simulink model "FM_V6_Zikun"  (R2022b)
settings: Solver=VariableStepAuto  StartTime=0.0  StopTime=1240
values from neighbouring files (symbols this model uses):
  A_fc = 550    [CNV.m]
  A_st = 1.1*A_fc*1E-4*n_cell*0.0012    (= 0.047553)    [CNV.m]
  A_T_rm = 0.005    [CNV.m]
  b11 = 0.005139    [CNV.m]
  b12 = 0.00326    [CNV.m]
  b2 = 350    [CNV.m]
  c1 = 10    [CNV.m]
  c3 = 2    [CNV.m]
  cc = 30    [CNV.m]
  Cd_rm = 0.0124    [CNV.m]
  Cp_air = 1005    [CNV.m]
  Cp_cl = 4180    [CNV.m]
  Cp_st = Cp_Al*1.5    (= 1350)    [CNV.m]
  F = 96485    [CNV.m]
  gamma = 1.4    [CNV.m]
  H_conv_st = 3    [CNV.m]
  i_max = 2.2    [CNV.m]
  k_ca_out = 0.2177*10^(-5)    (= 2.177e-06)    [CNV.m]
  K_sm_out = 0.3629*10^-5    (= 3.629e-06)    [CNV.m]
  kd_cp = 0.01    [CNV.m]
  kd_rm = 0    [CNV.m]
  ki_cp = 0.1    [CNV.m]
  ki_fan = -1E-5    (= -1e-05)    [CNV.m]
  ki_rm = -5E-8    (= -5e-08)    [CNV.m]
  kp_cp = 7.5    [CNV.m]
  kp_fan = -0.5    [CNV.m]
  kp_rm = -8E-7    (= -8e-07)    [CNV.m]
  M_a = 29*10^-3    (= 0.029)    [CNV.m]
  M_H2 = 2*10^-3    (= 0.002)    [CNV.m]
  m_H2_initial = P_atm*V_an/(R_H2*T_atm)    (= 0.00044494386048)    [CNV.m]
  m_H2O_initial = 0.005    [CNV.m]
  M_m_dry = 1.1    [CNV.m]
  M_N2 = 28*10^-3    (= 0.028)    [CNV.m]
  m_N2_initial = P_atm*(1-y_O2)*V_ca/(R_N2*T_atm)    (= 0.00586138039643)    [CNV.m]
  M_O2 = 32*10^-3    (= 0.032)    [CNV.m]
  m_O2_initial = P_atm*y_O2*V_ca/(R_O2*T_atm)    (= 0.00177998712422)    [CNV.m]
  m_st = n_cell*A_fc*t_m*rho_m_dry+(V_ca+V_an)*rho_Al*2.5    (= 87.4506875)    [CNV.m]
  M_v = 18*10^-3    (= 0.018)    [CNV.m]
  n_cell = 655    [CNV.m]
  P_a = P_atm*(1-L*h/T_atm)^(g*M_a/(R*L))    [CNV.m]
  P_atm = 101.25*10^3    (= 101250)    [CNV.m]
  P_ca_ref = 2.5*P_a    [CNV.m]
  phi_a = 0.1    [CNV.m]
  phi_des = 1    [CNV.m]
  R = 8.315    [CNV.m]
  R_a = 286.9    [CNV.m]
  R_H2 = 4124.3    [CNV.m]
  R_N2 = 296.8    [CNV.m]
  R_O2 = 259.8    [CNV.m]
  R_v = 461.5    [CNV.m]
  rho_a = P_a/(R_a*T_a)    [CNV.m]
  rho_H2 = 0.0899    [CNV.m]
  rho_m_dry = 0.002    [CNV.m]
  rho_N2 = 1.165    [CNV.m]
  T_a = T_atm-h*L    [CNV.m]
  T_atm = 298.15    [CNV.m]
  T_cl = 353.15    [CNV.m]
  t_m = 0.01    [CNV.m]
  T_rm = 303.15    [CNV.m]
  T_st_ref = 353.15    [CNV.m]
  V_an = n_cell*A_fc*10^(-4)*0.0005*0.3    (= 0.00540375)    [CNV.m]
  V_ca = n_cell*A_fc*10^(-4)*0.0006*0.3    (= 0.0064845)    [CNV.m]
  V_rm = 0.005    [CNV.m]
  V_sm = 0.02    [CNV.m]
  y_O2_ca_in = 0.21    [CNV.m]
libraries: fl_lib x64, nesl_utility x40, ee_lib x18, fl_ps_legacy_lib x6, SimscapeFluids_lib x5, slpidlib x4, simulink x3, batteryecm_lib x1, autolibshared x1
(part 4 of 6)

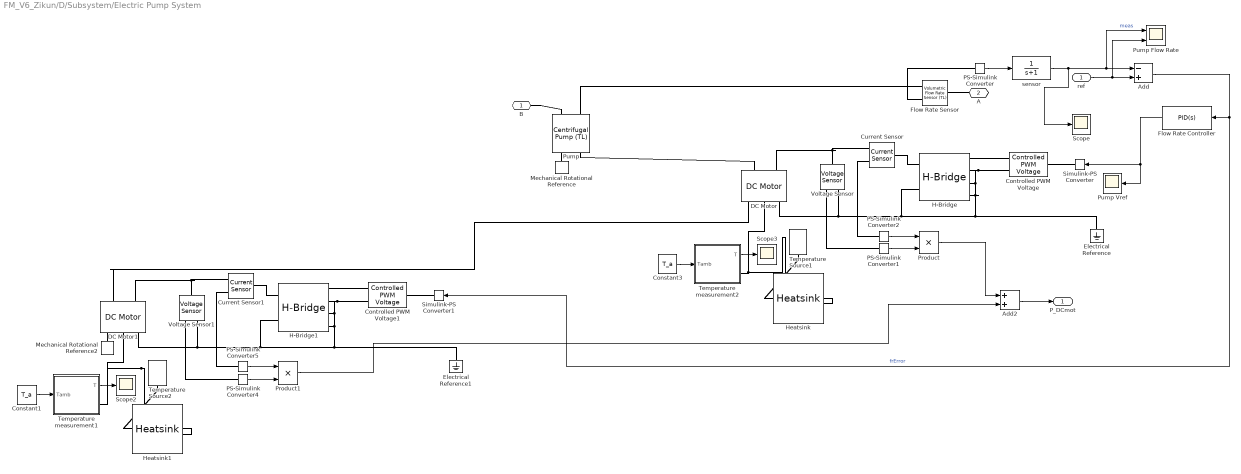
== system FM_V6_Zikun/D/Subsystem/Electric Pump System ==
  ref : Inport
  Add : Sum  Inputs=-+
  Add2 : Sum
  Constant1 : Constant  Value=T_a
  Constant3 : Constant  Value=T_a
  Controlled PWM Voltage : ee_lib/Integrated Circuits/Controlled PWM Voltage  F=4000 Hz  TD=0 s  pulse_width_offset=0 s  pulse_min=0 s  pwm_or_av=2  event_type=1  sample_time=5e-6 s  Vmin=0 V  Vmax=5 V  Vm=5 V  u_min=0  u_max=5
      settings: InternalSimscapePortConfiguration="{\"Bottom\":[],\"Left\":[{\"id\":\"u\",\"label\":\"u\",\"type\":\"input\"}],\"Right\":[{\"id\":\"p2\",\"label\":\"PWM\",\"type\":\"foundation.electrical.electrical\"},{\"id\":\"n2\",\"label\":\"REF\",\"type\":\"foundation.electrical.electrical\"}],\"Top\":[]}"
  Controlled PWM Voltage1 : ee_lib/Integrated Circuits/Controlled PWM Voltage  F=4000 Hz  TD=0 s  pulse_width_offset=0 s  pulse_min=0 s  pwm_or_av=2  event_type=1  sample_time=5e-6 s  Vmin=0 V  Vmax=5 V  Vm=5 V  u_min=0  u_max=5
      settings: InternalSimscapePortConfiguration="{\"Bottom\":[],\"Left\":[{\"id\":\"u\",\"label\":\"u\",\"type\":\"input\"}],\"Right\":[{\"id\":\"p2\",\"label\":\"PWM\",\"type\":\"foundation.electrical.electrical\"},{\"id\":\"n2\",\"label\":\"REF\",\"type\":\"foundation.electrical.electrical\"}],\"Top\":[]}"
  Current Sensor : fl_lib/Electrical/Electrical Sensors/Current Sensor
  Current Sensor1 : fl_lib/Electrical/Electrical Sensors/Current Sensor
  DC Motor : ee_lib/Electromechanical/Brushed Motors/DC Motor  Tag={'toolbox/physmod/elec/library/m/ee_lib_parts';'Electromechanical/Brushed_Motors/DC_Motor/Maxon/RE_65_388988_60.xml'}  field_option=ee.enum.field_option.pm  Rf=100 % Parameter not set Ohm  Lf=1 % Parameter not set H  Laf=0.15 % Parameter not set H  If0=0 % Parameter not set A  parameterization=ee.enum.dcparam_option.circuit_param  Ra=0.568 Ohm  La=0.251 mH  emf_or_torque=ee.enum.emf_or_torque.kv  Kv=16.05136 mV/rpm  Ki=153.27924 % Parameter estimated mN*m/A  T_stall=0.24e-3 % Parameter not set N*m  w_max=19100 % Parameter not set rpm  w_rated=15000 % Parameter not set rpm  P_rated=0.08 % Parameter not set W  V_rated=1.5 % Parameter not set V  lam_param=ee.enum.lam_param.current  i_noload=0.231 A  V_i_noload=60 V  J=1320 g*cm^2  lam=0 % % Parameter not set mN*m/(rad/s)  speed0=0 % Parameter not set rpm  enable_fault_armature=simscape.enum.onoff.off  rev_faulted=1 / 3 % Parameter not set  G_faulted_armature=1e-5 % Parameter not set S  fault_trigger_armature=ee.enum.faults.faultTrigger.temporal  t_fault_armature=1 % Parameter not set s  max_permissible_current_armature=inf % Parameter not set A  t_fail_on_current_armature=1 % Parameter not set s  enable_fault_field=simscape.enum.onoff.off  G_faulted_field=1e-5 % Parameter not set S  fault_trigger_field=ee.enum.faults.faultTrigger.temporal  t_fault_field=1 % Parameter not set s  max_permissible_current_field=inf % Parameter not set A  t_fail_on_current_field=1 % Parameter not set s  fault_action=simscape.enum.assert.action.none  alpha=3.93e-3 % Parameter not set 1/K  Tmeas=25 % Parameter not set degC  thermal_mass=667.588357588358 % Parameter estimated J/K  initial_temperature=25 % Parameter not set degC
      settings: AttributesFormatString=Maxon:RE_65_388988_60  InternalSimscapePortConfiguration="{\"Bottom\":[],\"Left\":[{\"id\":\"p\",\"label\":\"+\",\"type\":\"foundation.electrical.electrical\"},{\"id\":\"R\",\"label\":\"R\",\"type\":\"foundation.mechanical.rotational.rotational\"}],\"Right\":[{\"id\":\"n\",\"label\":\"-\",\"type\":\"foundation.electrical.electrical\"},{\"id\":\"H\",\"label\":\"H\",\"type\":\"foundation.thermal.thermal\"},{\"id\":\"C\",\"label\":\"C\",\"type\":\"foundation.mechanical.rotational.rotational\"}],\"Top\":[]}"
  DC Motor1 : ee_lib/Electromechanical/Brushed Motors/DC Motor  Tag={'toolbox/physmod/elec/library/m/ee_lib_parts';'Electromechanical/Brushed_Motors/DC_Motor/Maxon/RE_65_388988_60.xml'}  field_option=ee.enum.field_option.pm  Rf=100 % Parameter not set Ohm  Lf=1 % Parameter not set H  Laf=0.15 % Parameter not set H  If0=0 % Parameter not set A  parameterization=ee.enum.dcparam_option.circuit_param  Ra=0.568 Ohm  La=0.251 mH  emf_or_torque=ee.enum.emf_or_torque.kv  Kv=16.05136 mV/rpm  Ki=153.27924 % Parameter estimated mN*m/A  T_stall=0.24e-3 % Parameter not set N*m  w_max=19100 % Parameter not set rpm  w_rated=15000 % Parameter not set rpm  P_rated=0.08 % Parameter not set W  V_rated=1.5 % Parameter not set V  lam_param=ee.enum.lam_param.current  i_noload=0.231 A  V_i_noload=60 V  J=1320 g*cm^2  lam=0 % % Parameter not set mN*m/(rad/s)  speed0=0 % Parameter not set rpm  enable_fault_armature=simscape.enum.onoff.off  rev_faulted=1 / 3 % Parameter not set  G_faulted_armature=1e-5 % Parameter not set S  fault_trigger_armature=ee.enum.faults.faultTrigger.temporal  t_fault_armature=1 % Parameter not set s  max_permissible_current_armature=inf % Parameter not set A  t_fail_on_current_armature=1 % Parameter not set s  enable_fault_field=simscape.enum.onoff.off  G_faulted_field=1e-5 % Parameter not set S  fault_trigger_field=ee.enum.faults.faultTrigger.temporal  t_fault_field=1 % Parameter not set s  max_permissible_current_field=inf % Parameter not set A  t_fail_on_current_field=1 % Parameter not set s  fault_action=simscape.enum.assert.action.none  alpha=3.93e-3 % Parameter not set 1/K  Tmeas=25 % Parameter not set degC  thermal_mass=667.588357588358 % Parameter estimated J/K  initial_temperature=25 % Parameter not set degC
      settings: AttributesFormatString=Maxon:RE_65_388988_60  InternalSimscapePortConfiguration="{\"Bottom\":[],\"Left\":[{\"id\":\"p\",\"label\":\"+\",\"type\":\"foundation.electrical.electrical\"},{\"id\":\"R\",\"label\":\"R\",\"type\":\"foundation.mechanical.rotational.rotational\"}],\"Right\":[{\"id\":\"n\",\"label\":\"-\",\"type\":\"foundation.electrical.electrical\"},{\"id\":\"H\",\"label\":\"H\",\"type\":\"foundation.thermal.thermal\"},{\"id\":\"C\",\"label\":\"C\",\"type\":\"foundation.mechanical.rotational.rotational\"}],\"Top\":[]}"
  Electrical Reference : fl_lib/Electrical/Electrical Elements/Electrical Reference
  Electrical Reference1 : fl_lib/Electrical/Electrical Elements/Electrical Reference
  Flow Rate Sensor : fl_lib/Thermal Liquid/Sensors/Volumetric Flow Rate Sensor (TL)
      settings: InternalSimscapePortConfiguration="{\"Bottom\":[],\"Left\":[{\"id\":\"A\",\"label\":\"A\",\"type\":\"foundation.thermal_liquid.thermal_liquid\"}],\"Right\":[{\"id\":\"B\",\"label\":\"B\",\"type\":\"foundation.thermal_liquid.thermal_liquid\"},{\"id\":\"V\",\"label\":\"V\",\"type\":\"output\"}],\"Top\":[]}"
  Flow Rate Controller : slpidlib/PID Controller  Controller=PID  Form=Parallel  TimeDomain=Continuous-time  UseExternalTs=off  SampleTime=-1  IntegratorMethod=Forward Euler  FilterMethod=Forward Euler  ControllerParametersSource=internal  P=1  I=5e-1  UseKiTs=off  D=0  N=10  UseFilter=on  TunerSelectOption=Transfer Function Based (PID Tuner App)  ZeroCross=off  InitialConditionSource=internal  InitialConditionForIntegrator=0  InitialConditionForFilter=0  DifferentiatorICPrevScaledInput=0  ExternalReset=none  TrackingMode=off  Kt=1  LimitOutput=on  SatLimitsSource=internal  UpperSaturationLimit=5  LowerSaturationLimit=0  LinearizeAsGain=on  AntiWindupMode=none  Kb=1  LimitIntegrator=off  UpperIntegratorSaturationLimit=inf  LowerIntegratorSaturationLimit=-inf  POutMin=[]  POutMax=[]  IOutMin=[]  IOutMax=[]  DOutMin=[]  DOutMax=[]  NOutMin=[]  NOutMax=[]  SumOutMin=[]  SumOutMax=[]  SaturationOutMin=[]  SaturationOutMax=[]  PParamMin=[]  PParamMax=[]  IParamMin=[]  IParamMax=[]  DParamMin=[]  DParamMax=[]  NParamMin=[]  NParamMax=[]  KbParamMin=[]  KbParamMax=[]  KtParamMin=[]  KtParamMax=[]  KbOutMin=[]  KbOutMax=[]  KtOutMin=[]  KtOutMax=[]  IntegratorOutMin=[]  IntegratorOutMax=[]  FilterOutMin=[]  FilterOutMax=[]  SumI1OutMin=[]  SumI1OutMax=[]  SumI2OutMin=[]  SumI2OutMax=[]  SumI3OutMin=[]  SumI3OutMax=[]  SumI4OutMin=[]  SumI4OutMax=[]  SumDOutMin=[]  SumDOutMax=[]  DifferentiatorOutMin=[]  DifferentiatorOutMax=[]  FilterDiffOutCoefMin=[]  FilterDiffOutCoefMax=[]  ReciprocalOutMin=[]  ReciprocalOutMax=[]  SumDenOutMin=[]  SumDenOutMax=[]  SumNumOutMin=[]  SumNumOutMax=[]  DivideOutMin=[]  DivideOutMax=[]  UdiffTsProdOutMin=[]  UdiffTsProdOutMax=[]  NTsProdOutMin=[]  NTsProdOutMax=[]  UintegralTsProdOutMin=[]  UintegralTsProdOutMax=[]  UngainTsProdOutMin=[]  UngainTsProdOutMax=[]  ClampingZeroOutDataTypeStr=Inherit: Inherit via back propagation  ClampingZeroOutMin=[]  ClampingZeroOutMax=[]  FilterDenConstantOutDataTypeStr=Inherit: Inherit via back propagation  FilterDenConstantOutMin=[]  FilterDenConstantOutMax=[]  PCopyOutDataTypeStr=Inherit: Inherit via back propagation  PCopyOutMin=[]  PCopyOutMax=[]  NCopyOutDataTypeStr=Inherit: Inherit via back propagation  NCopyOutMin=[]  NCopyOutMax=[]  IntegratorContinuousStateAttributes=''  IntegratorStateMustResolveToSignalObject=off  IntegratorRTWStateStorageClass=Auto  FilterContinuousStateAttributes=''  FilterStateMustResolveToSignalObject=off  FilterRTWStateStorageClass=Auto  ParallelPVariant=InternalParameters  IdealPVariant=Disabled  IVariant=InternalParameters  DVariant=InternalParameters  IntegratorVariant=Continuous  SatVariant=Enabled  AWVariant=Passthrough  PCopyVariant=Disabled  TRVariant=Disabled  FdbkBlocksVariant=Forward  IdealPFdbkVariant=Disabled  SatFdbkVariant=Disabled  DerivativeFilterVariant=ContFilter  NVariant=InternalParameters  NCopyVariant=Disabled  FilterICVariant=InternalICsFilter  IntegratorICVariant=InternalICs  ExternalResetVariant=Disabled  TRSumVariant=Passthrough  SumFdbkVariant=Disabled  SumVariant=Sum_PID  TsampFilterVariant=InternalTs  TsampNgainVariant=Passthrough  TsampIntegralVariant=Passthrough  ExternalSaturationOutDataTypeStr=Inherit: Same as second input
  H-Bridge : ee_lib/Semiconductors & Converters/Converters/H-Bridge  supply_ports=ee.enum.supply_ports.hidesupply  pwm_or_av=2  regenerative_braking_mode=2  discontinuous=0  freewheeling_mode=1  Rload=3.38+0.1 Ohm  Lload=1e-5 H  F=4 kHz  Venable=2.5 V  Vmax=5 V  Vreverse=2.5 V  Vbrake=2.5 V  Vm=12 V  Ron=0.1 Ohm  Don=0.1 Ohm  Goff=1e-6 S  Tmeas=298.15 K  Ron2=0.1 Ohm  Don2=0.05 Ohm  Tmeas2=398.15 K  thermal_mass=100 J/K  initial_temperature=298.15 K
  H-Bridge1 : ee_lib/Semiconductors & Converters/Converters/H-Bridge  supply_ports=ee.enum.supply_ports.hidesupply  pwm_or_av=2  regenerative_braking_mode=2  discontinuous=0  freewheeling_mode=1  Rload=3.38+0.1 Ohm  Lload=1e-5 H  F=4 kHz  Venable=2.5 V  Vmax=5 V  Vreverse=2.5 V  Vbrake=2.5 V  Vm=12 V  Ron=0.1 Ohm  Don=0.1 Ohm  Goff=1e-6 S  Tmeas=298.15 K  Ron2=0.1 Ohm  Don2=0.05 Ohm  Tmeas2=398.15 K  thermal_mass=100 J/K  initial_temperature=298.15 K
  Heatsink : ee_lib/Passive/Thermal/Heatsink  parameterization=ee.enum.passive.thermal.heatsinkParam.rectangularFin  convection=ee.enum.passive.thermal.heatsinkConvection.natural  T_vec_Q=[10, 30, 50, 70, 90] K  v_vec_Q=[0, 1, 2, 3] m/s  Q_TLU1=[6.1, 23.6, 44.5, 67.5, 92.3] W  Q_TLU2=[6.1, 18.8, 22.8, 25.7; 23.6, 61.1, 73, 81.5; 44.5, 106.4, 125.9, 140.1; 67.5, 153.5, 180.7, 200.3; 92.3, 202.1, 236.9, 262] W  T_vec_h=[10, 30, 50, 70, 90] K  v_vec_h=[0, 1, 2, 3] m/s  h_TLU1=[5.4, 7.02, 7.98, 8.68, 9.26] W/(K*m^2)  h_TLU2=[5.4, 17.86, 22.17, 25.41; 7.02, 19.49, 23.8, 27.03; 7.97, 20.44, 24.75, 27.99; 8.68, 21.15, 25.46, 28.69; 9.26, 21.73, 26.04, 29.27] W/(K*m^2)  h_vec=[5, 10, 15, 20, 25, 30] W/(K*m^2)  eff_TLU=[96.97, 94.16, 91.53, 89.08, 86.78, 84.62]  height=0.1 m  thick=6.5e-4 m  depth=0.4 m  gap=9.4e-3 m  num_fins=100  k_fin=500 W/(K*m)  A_total=0.1171 m^2  nu=1.51e-5 m^2/s  alpha=2.07e-5 m^2/s  k_fluid=25e-3 W/(K*m)  beta=3.3e-3 1/K  mass=13 kg  sp_heat=550 J/(K*kg)  T_hs_specify=off  T_hs_priority=High  T_hs=300 K  T_hs_nominal_specify=off  T_hs_nominal_unit=K  T_hs_nominal_value=1  Q_A_specify=off  Q_A_priority=None  Q_A=0 W  Q_A_nominal_specify=off  Q_A_nominal_unit=W  Q_A_nominal_value=1  Q_C_specify=off  Q_C_priority=None  Q_C=0 W  Q_C_nominal_specify=off  Q_C_nominal_unit=W  Q_C_nominal_value=1
      settings: InternalSimscapePortConfiguration="{\"Bottom\":[{\"id\":\"C\",\"label\":\"C\",\"type\":\"foundation.thermal.thermal\"}],\"Left\":[],\"Right\":[],\"Top\":[{\"id\":\"A\",\"label\":\"A\",\"type\":\"foundation.thermal.thermal\"}]}"
  Heatsink1 : ee_lib/Passive/Thermal/Heatsink  parameterization=ee.enum.passive.thermal.heatsinkParam.rectangularFin  convection=ee.enum.passive.thermal.heatsinkConvection.natural  T_vec_Q=[10, 30, 50, 70, 90] K  v_vec_Q=[0, 1, 2, 3] m/s  Q_TLU1=[6.1, 23.6, 44.5, 67.5, 92.3] W  Q_TLU2=[6.1, 18.8, 22.8, 25.7; 23.6, 61.1, 73, 81.5; 44.5, 106.4, 125.9, 140.1; 67.5, 153.5, 180.7, 200.3; 92.3, 202.1, 236.9, 262] W  T_vec_h=[10, 30, 50, 70, 90] K  v_vec_h=[0, 1, 2, 3] m/s  h_TLU1=[5.4, 7.02, 7.98, 8.68, 9.26] W/(K*m^2)  h_TLU2=[5.4, 17.86, 22.17, 25.41; 7.02, 19.49, 23.8, 27.03; 7.97, 20.44, 24.75, 27.99; 8.68, 21.15, 25.46, 28.69; 9.26, 21.73, 26.04, 29.27] W/(K*m^2)  h_vec=[5, 10, 15, 20, 25, 30] W/(K*m^2)  eff_TLU=[96.97, 94.16, 91.53, 89.08, 86.78, 84.62]  height=0.1 m  thick=6.5e-4 m  depth=0.4 m  gap=9.4e-3 m  num_fins=100  k_fin=500 W/(K*m)  A_total=0.1171 m^2  nu=1.51e-5 m^2/s  alpha=2.07e-5 m^2/s  k_fluid=25e-3 W/(K*m)  beta=3.3e-3 1/K  mass=13 kg  sp_heat=550 J/(K*kg)  T_hs_specify=off  T_hs_priority=High  T_hs=300 K  T_hs_nominal_specify=off  T_hs_nominal_unit=K  T_hs_nominal_value=1  Q_A_specify=off  Q_A_priority=None  Q_A=0 W  Q_A_nominal_specify=off  Q_A_nominal_unit=W  Q_A_nominal_value=1  Q_C_specify=off  Q_C_priority=None  Q_C=0 W  Q_C_nominal_specify=off  Q_C_nominal_unit=W  Q_C_nominal_value=1
      settings: InternalSimscapePortConfiguration="{\"Bottom\":[{\"id\":\"C\",\"label\":\"C\",\"type\":\"foundation.thermal.thermal\"}],\"Left\":[],\"Right\":[],\"Top\":[{\"id\":\"A\",\"label\":\"A\",\"type\":\"foundation.thermal.thermal\"}]}"
  Mechanical Rotational Reference : fl_lib/Mechanical/Rotational Elements/Mechanical Rotational Reference
  Mechanical Rotational Reference2 : fl_lib/Mechanical/Rotational Elements/Mechanical Rotational Reference
  PS-Simulink Converter : nesl_utility/PS-Simulink Converter  PhysicalDomain=network_engine_domain  SubClassName=ps_output  LeftPortType=input  RightPortType=output  PseudoPeriodic=off  Frequencies=[]  VectorFormat=inherit  Unit=lpm  AffineConversion=off
  PS-Simulink Converter{1..2,4..5} (4 alike) : nesl_utility/PS-Simulink Converter  PhysicalDomain=network_engine_domain  SubClassName=ps_output  LeftPortType=input  RightPortType=output  PseudoPeriodic=off  Frequencies=[]  VectorFormat=inherit  Unit=inherit  AffineConversion=off
  Product : Product
  Product1 : Product
  Pump : SimscapeFluids_lib/Thermal Liquid/Pumps & Motors/Centrifugal Pump (TL)  pump_parameterization=fluids.thermal_liquid.pumps_motors.enum.CentrifugalPumpParameterization.Table1D  capacity_ref_nominal=7 lpm  head_ref_nominal=3 m  power_ref_nominal=5 W  head_ref_max=4 m  capacity_ref_max=12 lpm  omega_ref_analytic=4000 rpm  flow_rate_1D_TLU=[16.67, 30, 40, 53.33, 66.67, 83.33] lpm  head_1D_TLU=[50, 47.5, 45, 40, 35, 25] m  power_1D_TLU=[.6, .75, .85, .93, .98, .99] kW  omega_ref_1D=3500 rpm  rho_ref_1D=998.21 kg/m^3  flow_rate_2D_TLU=[16.67, 23.33, 30, 40, 53.33, 60] lpm  omega_2D_TLU=[2450, 2800, 3150, 3500] rpm  head_2D_TLU=[25, 32.7, 42.5, 50; 24, 31.7, 41, 49; 22.7, 30.5, 39, 47.5; 20, 28, 36, 45; 15.7, 24, 32, 40; 12.5, 21, 29.5, 37.5] m  power_2D_TLU=[.28, .38, .5, .6; .31, .41, .55, .68; .33, .44, .6, .75; .36, .48, .65, .83; .38, .53, .72, .93; .39, .55, .75, .97] kW  rho_ref_2D=998.21 kg/m^3  diameter_ratio=1  mech_orientation=fluids.thermal_liquid.pumps_motors.enum.CentrifugalPumpMechOrientation.Positive  area=0.03^2*pi/4 m^2
      settings: InternalSimscapePortConfiguration="{\"Bottom\":[],\"Left\":[{\"id\":\"A\",\"label\":\"A\",\"type\":\"foundation.thermal_liquid.thermal_liquid\"},{\"id\":\"B\",\"label\":\"B\",\"type\":\"foundation.thermal_liquid.thermal_liquid\"}],\"Right\":[{\"id\":\"R\",\"label\":\"R\",\"type\":\"foundation.mechanical.rotational.rotational\"},{\"id\":\"C\",\"label\":\"C\",\"type\":\"foundation.mechanical.rotational.rotational\"}],\"Top\":[]}"
  Pump Flow Rate : Scope  NumInputPorts=2
  Pump Vref : Scope
  Scope : Scope
  Scope2 : Scope
  Scope3 : Scope
  Simulink-PS Converter : nesl_utility/Simulink-PS Converter  PhysicalDomain=network_engine_domain  SubClassName=ps_input  LeftPortType=input  RightPortType=output  PseudoPeriodic=off  Frequencies=[]  NoiseDistribution=none  NoiseParameters=[]  Unit=1  AffineConversion=off  FilteringAndDerivatives=provide  SimscapeFilterOrder=1  InputFilterTimeConstant=0.001  UdotUserProvided=0
  Simulink-PS Converter1 : nesl_utility/Simulink-PS Converter  PhysicalDomain=network_engine_domain  SubClassName=ps_input  LeftPortType=input  RightPortType=output  PseudoPeriodic=off  Frequencies=[]  NoiseDistribution=none  NoiseParameters=[]  Unit=1  AffineConversion=off  FilteringAndDerivatives=provide  SimscapeFilterOrder=1  InputFilterTimeConstant=0.001  UdotUserProvided=0
  Temperature measurement1 : Subsystem
  Temperature measurement2 : Subsystem
  Temperature Source1 : fl_lib/Thermal/Thermal Sources/Temperature Source  temperature=T_a K
  Temperature Source2 : fl_lib/Thermal/Thermal Sources/Temperature Source  temperature=T_a K
  Voltage Sensor : fl_lib/Electrical/Electrical Sensors/Voltage Sensor
  Voltage Sensor1 : fl_lib/Electrical/Electrical Sensors/Voltage Sensor
  sensor : TransferFcn  Denominator=[1, 1]
  B : PMIOPort  Side=Left
  A : PMIOPort  Port=2  Side=Left
  P_DCmot : Outport
  wires:
  Flow Rate Controller/1 -> Pump Vref/1, Simulink-PS Converter/1
  Add/1 -> Simulink-PS Converter1/1, Flow Rate Controller/1  "frError"
  PS-Simulink Converter/1 -> sensor/1
  sensor/1 -> Scope/1, Pump Flow Rate/1, Add/1  "meas"
  PS-Simulink Converter2/1 -> Product/1
  PS-Simulink Converter1/1 -> Product/2
  Product/1 -> Add2/1
  Temperature measurement2/1(T) -> Scope3/1
  Constant3/1 -> Temperature measurement2/1(Tamb)
  Product1/1 -> Add2/2
  PS-Simulink Converter4/1 -> Product1/2
  Temperature measurement1/1(T) -> Scope2/1
  ref/1 -> Pump Flow Rate/2, Add/2
  PS-Simulink Converter5/1 -> Product1/1
  Constant1/1 -> Temperature measurement1/1(Tamb)
  Add2/1 -> P_DCmot/1
  connections:
  Mechanical Rotational Reference/LConn1 -- Pump/RConn2
  DC Motor/LConn2 -- Pump/RConn1
  B/RConn1 -- Pump/LConn2
  H-Bridge/LConn4 -- Controlled PWM Voltage/RConn2 -- H-Bridge/LConn2 -- H-Bridge/LConn3 -- DC Motor/RConn1 -- Voltage Sensor/RConn2 -- H-Bridge/RConn2 -- Electrical Reference/LConn1
  H-Bridge/LConn1 -- Controlled PWM Voltage/RConn1
  Voltage Sensor/LConn1 -- DC Motor/LConn1 -- Current Sensor/RConn2
  Flow Rate Sensor/LConn1 -- A/RConn1
  Flow Rate Sensor/RConn1 -- Pump/LConn1
  Flow Rate Sensor/RConn2 -- PS-Simulink Converter/LConn1
  Simulink-PS Converter/RConn1 -- Controlled PWM Voltage/LConn1
  PS-Simulink Converter1/LConn1 -- Voltage Sensor/RConn1
  PS-Simulink Converter2/LConn1 -- Current Sensor/RConn1
  Current Sensor/LConn1 -- H-Bridge/RConn1
  DC Motor/RConn3 -- DC Motor1/LConn2
  Temperature measurement2/RConn1 -- DC Motor/RConn2 -- Heatsink/RConn1
  Heatsink/LConn1 -- Temperature Source1/LConn1
  Current Sensor1/RConn2 -- Voltage Sensor1/LConn1 -- DC Motor1/LConn1
  Heatsink1/RConn1 -- Temperature measurement1/RConn1 -- DC Motor1/RConn2
  H-Bridge1/LConn2 -- H-Bridge1/LConn4 -- DC Motor1/RConn1 -- Voltage Sensor1/RConn2 -- H-Bridge1/RConn2 -- Electrical Reference1/LConn1 -- H-Bridge1/LConn3 -- Controlled PWM Voltage1/RConn2
  Heatsink1/LConn1 -- Temperature Source2/LConn1
  Simulink-PS Converter1/RConn1 -- Controlled PWM Voltage1/LConn1
  PS-Simulink Converter4/LConn1 -- Voltage Sensor1/RConn1
  Current Sensor1/LConn1 -- H-Bridge1/RConn1
  PS-Simulink Converter5/LConn1 -- Current Sensor1/RConn1
  H-Bridge1/LConn1 -- Controlled PWM Voltage1/RConn1
  DC Motor1/RConn3 -- Mechanical Rotational Reference2/LConn1

== system FM_V6_Zikun/D/Subsystem/Temperature measurement ==
  Tamb : Inport
  Convective Heat Transfer : fl_lib/Thermal/Thermal Elements/Convective Heat Transfer  thermal_type=foundation.enum.constant_variable.constant  area=0.1 m^2  heat_tr_coeff=5 W/(m^2 * K)  min_heat_tr_coeff=1e-3 W/(K*m^2)  T_specify=off  T_priority=None  T=0 K  T_nominal_specify=off  T_nominal_unit=K  T_nominal_value=1  Q_specify=off  Q_priority=None  Q=0 J/s  Q_nominal_specify=off  Q_nominal_unit=J/s  Q_nominal_value=1
  PS-Simulink Converter1 : nesl_utility/PS-Simulink Converter  PhysicalDomain=network_engine_domain  SubClassName=ps_output  LeftPortType=input  RightPortType=output  PseudoPeriodic=off  Frequencies=[]  VectorFormat=1-D array  Unit=degC  AffineConversion=on
  Simulink-PS Converter1 : nesl_utility/Simulink-PS Converter  PhysicalDomain=network_engine_domain  SubClassName=ps_input  LeftPortType=input  RightPortType=output  PseudoPeriodic=off  Frequencies=[]  NoiseDistribution=none  NoiseParameters=[]  Unit=degC  AffineConversion=on  FilteringAndDerivatives=zero  SimscapeFilterOrder=1  InputFilterTimeConstant=0.001  UdotUserProvided=1
  Temperature Sensor : fl_lib/Thermal/Thermal Sensors/Temperature Sensor
  Temperature Source : fl_lib/Thermal/Thermal Sources/Controlled Temperature Source
  Thermal Reference : fl_lib/Thermal/Thermal Elements/Thermal Reference
  H : PMIOPort  Side=Right
  T : Outport  VectorParamsAs1DForOutWhenUnconnected=off
  wires:
  Tamb/1 -> Simulink-PS Converter1/1
  PS-Simulink Converter1/1 -> T/1  "Temperature [degC]"
  connections:
  Convective Heat Transfer/RConn1 -- Temperature Source/LConn1
  Temperature Sensor/RConn2 -- PS-Simulink Converter1/LConn1
  Temperature Sensor/LConn1 -- H/RConn1 -- Convective Heat Transfer/LConn1
  Simulink-PS Converter1/RConn1 -- Temperature Source/RConn1
  Thermal Reference/LConn1 -- Temperature Sensor/RConn1 -- Temperature Source/RConn2

== system FM_V6_Zikun/D/Subsystem/Temperature measurement1 ==
  Tamb : Inport
  Convective Heat Transfer : fl_lib/Thermal/Thermal Elements/Convective Heat Transfer  thermal_type=foundation.enum.constant_variable.constant  area=0.1 m^2  heat_tr_coeff=5 W/(m^2 * K)  min_heat_tr_coeff=1e-3 W/(K*m^2)  T_specify=off  T_priority=None  T=0 K  T_nominal_specify=off  T_nominal_unit=K  T_nominal_value=1  Q_specify=off  Q_priority=None  Q=0 J/s  Q_nominal_specify=off  Q_nominal_unit=J/s  Q_nominal_value=1
  PS-Simulink Converter1 : nesl_utility/PS-Simulink Converter  PhysicalDomain=network_engine_domain  SubClassName=ps_output  LeftPortType=input  RightPortType=output  PseudoPeriodic=off  Frequencies=[]  VectorFormat=1-D array  Unit=degC  AffineConversion=on
  Simulink-PS Converter1 : nesl_utility/Simulink-PS Converter  PhysicalDomain=network_engine_domain  SubClassName=ps_input  LeftPortType=input  RightPortType=output  PseudoPeriodic=off  Frequencies=[]  NoiseDistribution=none  NoiseParameters=[]  Unit=degC  AffineConversion=on  FilteringAndDerivatives=zero  SimscapeFilterOrder=1  InputFilterTimeConstant=0.001  UdotUserProvided=1
  Temperature Sensor : fl_lib/Thermal/Thermal Sensors/Temperature Sensor
  Temperature Source : fl_lib/Thermal/Thermal Sources/Controlled Temperature Source
  Thermal Reference : fl_lib/Thermal/Thermal Elements/Thermal Reference
  H : PMIOPort  Side=Right
  T : Outport  VectorParamsAs1DForOutWhenUnconnected=off
  wires:
  Tamb/1 -> Simulink-PS Converter1/1
  PS-Simulink Converter1/1 -> T/1  "Temperature [degC]"
  connections:
  Convective Heat Transfer/RConn1 -- Temperature Source/LConn1
  Temperature Sensor/RConn2 -- PS-Simulink Converter1/LConn1
  Temperature Sensor/LConn1 -- H/RConn1 -- Convective Heat Transfer/LConn1
  Simulink-PS Converter1/RConn1 -- Temperature Source/RConn1
  Thermal Reference/LConn1 -- Temperature Sensor/RConn1 -- Temperature Source/RConn2

== system FM_V6_Zikun/D/Subsystem/Temperature measurement2 ==
  Tamb : Inport
  Convective Heat Transfer : fl_lib/Thermal/Thermal Elements/Convective Heat Transfer  thermal_type=foundation.enum.constant_variable.constant  area=0.1 m^2  heat_tr_coeff=5 W/(m^2 * K)  min_heat_tr_coeff=1e-3 W/(K*m^2)  T_specify=off  T_priority=None  T=0 K  T_nominal_specify=off  T_nominal_unit=K  T_nominal_value=1  Q_specify=off  Q_priority=None  Q=0 J/s  Q_nominal_specify=off  Q_nominal_unit=J/s  Q_nominal_value=1
  PS-Simulink Converter1 : nesl_utility/PS-Simulink Converter  PhysicalDomain=network_engine_domain  SubClassName=ps_output  LeftPortType=input  RightPortType=output  PseudoPeriodic=off  Frequencies=[]  VectorFormat=1-D array  Unit=degC  AffineConversion=on
  Simulink-PS Converter1 : nesl_utility/Simulink-PS Converter  PhysicalDomain=network_engine_domain  SubClassName=ps_input  LeftPortType=input  RightPortType=output  PseudoPeriodic=off  Frequencies=[]  NoiseDistribution=none  NoiseParameters=[]  Unit=degC  AffineConversion=on  FilteringAndDerivatives=zero  SimscapeFilterOrder=1  InputFilterTimeConstant=0.001  UdotUserProvided=1
  Temperature Sensor : fl_lib/Thermal/Thermal Sensors/Temperature Sensor
  Temperature Source : fl_lib/Thermal/Thermal Sources/Controlled Temperature Source
  Thermal Reference : fl_lib/Thermal/Thermal Elements/Thermal Reference
  H : PMIOPort  Side=Right
  T : Outport  VectorParamsAs1DForOutWhenUnconnected=off
  wires:
  Tamb/1 -> Simulink-PS Converter1/1
  PS-Simulink Converter1/1 -> T/1  "Temperature [degC]"
  connections:
  Convective Heat Transfer/RConn1 -- Temperature Source/LConn1
  Temperature Sensor/RConn2 -- PS-Simulink Converter1/LConn1
  Temperature Sensor/LConn1 -- H/RConn1 -- Convective Heat Transfer/LConn1
  Simulink-PS Converter1/RConn1 -- Temperature Source/RConn1
  Thermal Reference/LConn1 -- Temperature Sensor/RConn1 -- Temperature Source/RConn2

== system FM_V6_Zikun/D/Subsystem/Temperature measurement3 ==
  Tamb : Inport
  Convective Heat Transfer : fl_lib/Thermal/Thermal Elements/Convective Heat Transfer  thermal_type=foundation.enum.constant_variable.constant  area=0.1 m^2  heat_tr_coeff=5 W/(m^2 * K)  min_heat_tr_coeff=1e-3 W/(K*m^2)  T_specify=off  T_priority=None  T=0 K  T_nominal_specify=off  T_nominal_unit=K  T_nominal_value=1  Q_specify=off  Q_priority=None  Q=0 J/s  Q_nominal_specify=off  Q_nominal_unit=J/s  Q_nominal_value=1
  PS-Simulink Converter1 : nesl_utility/PS-Simulink Converter  PhysicalDomain=network_engine_domain  SubClassName=ps_output  LeftPortType=input  RightPortType=output  PseudoPeriodic=off  Frequencies=[]  VectorFormat=1-D array  Unit=degC  AffineConversion=on
  Simulink-PS Converter1 : nesl_utility/Simulink-PS Converter  PhysicalDomain=network_engine_domain  SubClassName=ps_input  LeftPortType=input  RightPortType=output  PseudoPeriodic=off  Frequencies=[]  NoiseDistribution=none  NoiseParameters=[]  Unit=degC  AffineConversion=on  FilteringAndDerivatives=zero  SimscapeFilterOrder=1  InputFilterTimeConstant=0.001  UdotUserProvided=1
  Temperature Sensor : fl_lib/Thermal/Thermal Sensors/Temperature Sensor
  Temperature Source : fl_lib/Thermal/Thermal Sources/Controlled Temperature Source
  Thermal Reference : fl_lib/Thermal/Thermal Elements/Thermal Reference
  H : PMIOPort  Side=Right
  T : Outport  VectorParamsAs1DForOutWhenUnconnected=off
  wires:
  Tamb/1 -> Simulink-PS Converter1/1
  PS-Simulink Converter1/1 -> T/1  "Temperature [degC]"
  connections:
  Convective Heat Transfer/RConn1 -- Temperature Source/LConn1
  Temperature Sensor/RConn2 -- PS-Simulink Converter1/LConn1
  Temperature Sensor/LConn1 -- H/RConn1 -- Convective Heat Transfer/LConn1
  Simulink-PS Converter1/RConn1 -- Temperature Source/RConn1
  Thermal Reference/LConn1 -- Temperature Sensor/RConn1 -- Temperature Source/RConn2

== system FM_V6_Zikun/Subsystem/Compressor/Power calc 2 ==
  P_cp_out : Inport
  P_cp_in : Inport  Port=2
  gamma : Inport  Port=3
  W_cp_in : Inport  Port=4
  Constant2 : Constant  Value=rho_a
  Divide : Product  Inputs=*/
  MATLAB Function : MATLAB Function  TreatAsAtomicUnit=on
  Scope : Scope
  Power_cp : Outport
  wires:
  P_cp_out/1 -> Divide/1
  gamma/1 -> MATLAB Function/1(gamma)
  P_cp_in/1 -> MATLAB Function/2(P_cp_in), Divide/2
  W_cp_in/1 -> MATLAB Function/3(W_ca_in)
  Constant2/1 -> MATLAB Function/4(rho_a)
  MATLAB Function/1(Power_cp) -> Power_cp/1
  Divide/1 -> Scope/1, MATLAB Function/5(copratio)

== system FM_V6_Zikun/Subsystem/Compressor/Subsystem ==
  W_O2_ca_in : Inport
  I_st : Inport  Port=2
  P_ca : Inport  Port=3
  Add : Sum  Inputs=+-
  Add1 : Sum  Inputs=+++++
  Constant : Constant  Value=T_a
  Constant1 : Constant  Value=phi_a
  Constant2 : Constant  Value=M_v
  Constant3 : Constant  Value=y_O2_ca_in
  Constant4 : Constant  Value=n_cell
  Constant5 : Constant  Value=F
  Constant6 : Constant  Value=P_a
  Constant7 : Constant  Value=M_a
  Constant8 : Constant  Value=M_O2
  Derivative : Derivative
  Gain : Gain  Gain=kp_cp
  Gain1 : Gain  Gain=ki_cp
  Gain2 : Gain  Gain=1/0.21
  Gain3 : Gain  Gain=kd_cp
  Integrator : Integrator
  MATLAB Function : MATLAB Function  TreatAsAtomicUnit=on
  Subsystem1 : Subsystem  Commented=on
  oer : Constant  Value=2
  W_cp : Outport
  wires:
  Constant7/1 -> MATLAB Function/10(M_a_ca_in)
  Constant3/1 -> MATLAB Function/8(y_O2_ca_in)
  Constant5/1 -> MATLAB Function/7(F)
  Constant4/1 -> MATLAB Function/6(n_cell)
  I_st/1 -> MATLAB Function/5(I_st)
  oer/1 -> MATLAB Function/9(O2_ER)
  Constant6/1 -> MATLAB Function/3(P_cp_in)
  Constant/1 -> MATLAB Function/4(T_cp_in)
  Constant1/1 -> MATLAB Function/2(phi_a)
  Constant2/1 -> MATLAB Function/1(M_v)
  W_O2_ca_in/1 -> Add/2
  MATLAB Function/2(W_O2_ref) -> Add/1
  Gain/1 -> Add1/2
  Add1/1 -> W_cp/1
  MATLAB Function/1(W_cp) -> Add1/1
  Constant8/1 -> MATLAB Function/11(M_O2)
  Integrator/1 -> Gain1/1
  Gain1/1 -> Add1/3
  Gain2/1 -> Gain/1, Integrator/1, Derivative/1
  Add/1 -> Gain2/1
  Derivative/1 -> Gain3/1
  Gain3/1 -> Add1/4
  Subsystem1/1(diff) -> Add1/5
  P_ca/1 -> Subsystem1/1(P_ca)

== system FM_V6_Zikun/Subsystem/Compressor/Temperature of the air leaving the compressor (2.8) ==
  T_atm : Inport
  eta_cp : Inport  Port=2
  P_sm : Inport  Port=3
  P_atm : Inport  Port=4
  gamma : Inport  Port=5
  Add : Sum
  Gain calc : MATLAB Function  TreatAsAtomicUnit=on
  Scope : Scope
  Temperature add : MATLAB Function  TreatAsAtomicUnit=on
  T_cp_out : Outport
  wires:
  gamma/1 -> Gain calc/1(gamma)
  T_atm/1 -> Add/1, Temperature add/1(T_atm)
  eta_cp/1 -> Temperature add/2(eta_cp)
  P_sm/1 -> Temperature add/3(P_sm)
  P_atm/1 -> Temperature add/4(P_atm)
  Temperature add/1(T_add_cp) -> Add/2
  Add/1 -> T_cp_out/1
  Gain calc/1(gamma_gain) -> Scope/1, Temperature add/5(gamma_gain)

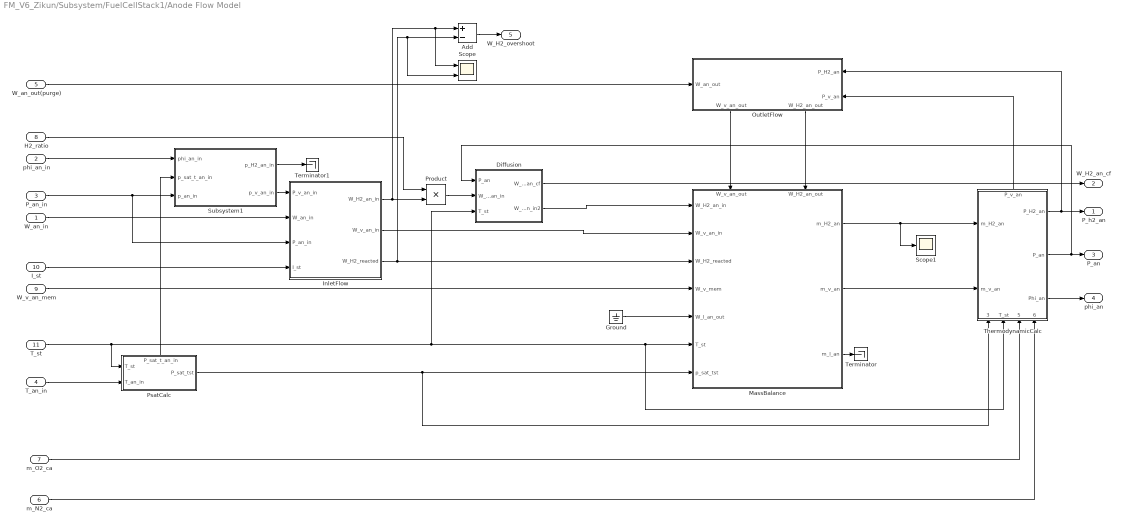
== system FM_V6_Zikun/Subsystem/FuelCellStack1/Anode Flow Model ==
  W_an_in : Inport
  phi_an_in : Inport  Port=2
  P_an_in : Inport  Port=3
  T_an_in : Inport  Port=4
  W_an_out(purge) : Inport  Port=5
  m_N2_ca : Inport  Port=6
  m_O2_ca : Inport  Port=7
  H2_ratio : Inport  Port=8
  W_v_an_mem : Inport  Port=9
  I_st : Inport  Port=10
  T_st : Inport  Port=11
  Add : Sum  Inputs=+-
  Diffusion : Subsystem
  Ground : Ground
  InletFlow : Subsystem
  MassBalance : Subsystem
      settings: PortSchema="{\"entries\":[{\"content\":{\"sides\":[{\"content\":{\"connectorIds\":[\"In1\",\"In2\",\"In3\",\"In4\",\"In5\",\"In6\",\"In7\"]},\"type\":\"ConnectorPlacement.EquallySpacedRectSide\",\"uuid\":\"47913980-4837-4670-9a70-20a28a5e1cf6\"},{\"content\":{\"connectorIds\":[\"Out1\",\"Out2\",\"Out3\"],\"side\":\"RIGHT\"},\"type\":\"ConnectorPlacement.EquallySpacedRectSide\",\"uuid\":\"6e1f0fd0-09cf-4914-9f02-3e28247eab40\"},{\"content\":{\"connectorIds\":[\"In8\",\"In9\"],\"side\":\"TOP\"},\"type\":\"ConnectorPlacement.EquallySpacedRectSide\",\"uuid\":\"fdbbf9ee-836e-4b74-8c8b-93bb1660498f\"},{\"content\":{\"connectorIds\":[],\"side\":\"BOTTOM\"},\"type\":\"ConnectorPlacement.EquallySpacedRectSide\",\"uuid\":\"f9503325-eb72-4272-af06-2ab6d07ae2a1\"}]},\"type\":\"ConnectorPlacement.EquallySpacedConnector\",\"uuid\":\"b1cb0204-eb42-499b-8aff-5daf38dba684\"}],\"packageUris\":[\"http://schema.mathworks.com/mf0/Connector/R2020b\"],\"version\":\"1.0\"}"
  OutletFlow : Subsystem
      settings: PortSchema="{\"entries\":[{\"content\":{\"sides\":[{\"content\":{\"connectorIds\":[\"In1\"]},\"type\":\"ConnectorPlacement.EquallySpacedRectSide\",\"uuid\":\"a22c9b48-231f-4509-82e5-8f3ee39292f2\"},{\"content\":{\"connectorIds\":[\"In2\",\"In3\"],\"side\":\"RIGHT\"},\"type\":\"ConnectorPlacement.EquallySpacedRectSide\",\"uuid\":\"e209ca62-0ee1-4f06-871f-c25c9d944ffa\"},{\"content\":{\"connectorIds\":[],\"side\":\"TOP\"},\"type\":\"ConnectorPlacement.EquallySpacedRectSide\",\"uuid\":\"93a24582-fa3f-4fb5-a9f4-6caa7b20623d\"},{\"content\":{\"connectorIds\":[\"Out1\",\"Out2\"],\"side\":\"BOTTOM\"},\"type\":\"ConnectorPlacement.EquallySpacedRectSide\",\"uuid\":\"04b659a5-3d39-499b-aa02-9d7b346de914\"}]},\"type\":\"ConnectorPlacement.EquallySpacedConnector\",\"uuid\":\"7b887b26-af8b-4a52-ae26-1ee7ea24304c\"}],\"packageUris\":[\"http://schema.mathworks.com/mf0/Connector/R2020b\"],\"version\":\"1.0\"}"
  Product : Product
  PsatCalc : Subsystem
      settings: PortSchema="{\"entries\":[{\"content\":{\"sides\":[{\"content\":{\"connectorIds\":[\"In1\",\"In2\"]},\"type\":\"ConnectorPlacement.EquallySpacedRectSide\",\"uuid\":\"eb5b356c-3a72-4d67-b4c5-4dc1b428f129\"},{\"content\":{\"connectorIds\":[\"Out1\"],\"side\":\"RIGHT\"},\"type\":\"ConnectorPlacement.EquallySpacedRectSide\",\"uuid\":\"0cc1be20-8d19-4c9e-8406-f1a101e38c53\"},{\"content\":{\"connectorIds\":[\"Out2\"],\"side\":\"TOP\"},\"type\":\"ConnectorPlacement.EquallySpacedRectSide\",\"uuid\":\"9b69fe96-957d-4053-a8ad-90651bf4754f\"}]},\"type\":\"ConnectorPlacement.EquallySpacedConnector\",\"uuid\":\"56b0af2c-dae1-4adc-b708-26ac7c8a2b07\"}],\"packageUris\":[\"http://schema.mathworks.com/mf0/Connector/R2020b\"],\"version\":\"1.0\"}"
  Scope : Scope  NumInputPorts=2
  Scope1 : Scope
  Subsystem1 : Subsystem
  Terminator : Terminator
  Terminator1 : Terminator
  ThermodynamicCalc : Subsystem
      settings: PortSchema="{\"entries\":[{\"content\":{\"sides\":[{\"content\":{\"connectorIds\":[\"In1\",\"In2\"]},\"type\":\"ConnectorPlacement.EquallySpacedRectSide\",\"uuid\":\"1ac3cd26-c6f9-4678-a43b-89d74228e3da\"},{\"content\":{\"connectorIds\":[\"Out1\",\"Out2\",\"Out3\"],\"side\":\"RIGHT\"},\"type\":\"ConnectorPlacement.EquallySpacedRectSide\",\"uuid\":\"e8374325-0971-4eae-996c-945c49276d1a\"},{\"content\":{\"connectorIds\":[\"Out4\"],\"side\":\"TOP\"},\"type\":\"ConnectorPlacement.EquallySpacedRectSide\",\"uuid\":\"e1484837-f333-492b-af5c-11e40db9a824\"},{\"content\":{\"connectorIds\":[\"In3\",\"In4\",\"In5\",\"In6\"],\"side\":\"BOTTOM\"},\"type\":\"ConnectorPlacement.EquallySpacedRectSide\",\"uuid\":\"5a4b2b1f-75b1-4978-afa9-3cc7ca4083b5\"}]},\"type\":\"ConnectorPlacement.EquallySpacedConnector\",\"uuid\":\"58e29f0f-5a8f-42b3-8c0c-a4515a273d1c\"}],\"packageUris\":[\"http://schema.mathworks.com/mf0/Connector/R2020b\"],\"version\":\"1.0\"}"
  P_h2_an : Outport
  W_H2_an_cf : Outport  Port=2
  P_an : Outport  Port=3
  phi_an : Outport  Port=4
  W_H2_overshoot : Outport  Port=5
  wires:
  OutletFlow/1(W_v_an_out) -> MassBalance/8(W_v_an_out)
  MassBalance/2(m_v_an) -> ThermodynamicCalc/2(m_v_an)
  ThermodynamicCalc/1(P_H2_an) -> P_h2_an/1, OutletFlow/2(P_H2_an)
  ThermodynamicCalc/4(P_v_an) -> OutletFlow/3(P_v_an)
  Subsystem1/2(p_v_an_in) -> InletFlow/1(P_v_an_in)
  InletFlow/2(W_v_an_in) -> MassBalance/2(W_v_an_in)
  W_an_in/1 -> InletFlow/2(W_an_in)
  Ground/1 -> MassBalance/5(W_l_an_out)
  W_v_an_mem/1 -> MassBalance/4(W_v_mem)
  phi_an_in/1 -> Subsystem1/1(phi_an_in)
  P_an_in/1 -> InletFlow/3(P_an_in), Subsystem1/3(p_an_in)
  PsatCalc/2(P_sat_t_an_in) -> Subsystem1/2(p_sat_t_an_in)
  T_an_in/1 -> PsatCalc/2(T_an_in)
  I_st/1 -> InletFlow/4(I_st)
  MassBalance/3(m_l_an) -> Terminator/1
  T_st/1 -> PsatCalc/1(T_st), Diffusion/3(T_st), MassBalance/6(T_st), ThermodynamicCalc/4(T_st)
  PsatCalc/1(P_sat_tst) -> ThermodynamicCalc/3(P_sat(T_st)), MassBalance/7(p_sat_tst)
  ThermodynamicCalc/3(Phi_an) -> phi_an/1
  Subsystem1/1(p_H2_an_in) -> Terminator1/1
  Diffusion/2(W_H2_an_in2) -> MassBalance/1(W_H2_an_in)
  OutletFlow/2(W_H2_an_out) -> MassBalance/9(W_H2_an_out)
  Diffusion/1(W_H2_an_cf) -> W_H2_an_cf/1
  InletFlow/1(W_H2_an_in) -> Scope/1, Add/1, Product/2
  MassBalance/1(m_H2_an) -> Scope1/1, ThermodynamicCalc/1(m_H2_an)
  H2_ratio/1 -> Product/1
  InletFlow/3(W_H2_reacted) -> Scope/2, Add/2, MassBalance/3(W_H2_reacted)
  W_an_out(purge)/1 -> OutletFlow/1(W_an_out)
  m_O2_ca/1 -> ThermodynamicCalc/5(m_O2_an)
  m_N2_ca/1 -> ThermodynamicCalc/6(m_N2_an)
  Product/1 -> Diffusion/2(W_H2_an_in)
  ThermodynamicCalc/2(P_an) -> P_an/1, Diffusion/1(P_an)
  Add/1 -> W_H2_overshoot/1

== system FM_V6_Zikun/Subsystem/FuelCellStack1/Anode Recirculation and Purge System1 ==
  T_an : Inport
  P_an : Inport  Port=2
  W_O2_ca_cf : Inport  Port=3
  W_N2_ca_cf : Inport  Port=4
  Add3 : Sum
  Constant : Constant  Value=R_N2
  Constant1 : Constant  Value=R_O2
  Constant2 : Constant  Value=V_an
  Gain : Gain
  Gain1 : Gain
  Integrator : Integrator  ExternalReset=rising
  Integrator1 : Integrator  ExternalReset=rising
  MATLAB Function : MATLAB Function  TreatAsAtomicUnit=on
  MATLAB Function1 : MATLAB Function  TreatAsAtomicUnit=on
  Pipe Volume : Constant  Value=0.001
  Pulse Generator : DiscretePulseGenerator  PulseType=Time based  Period=60
  Scope : Scope
  Scope1 : Scope
  Scope2 : Scope  NumInputPorts=2
  H2_ratio : Outport
  m_O2_ca : Outport  Port=2
  m_N2_ca : Outport  Port=3
  wires:
  W_N2_ca_cf/1 -> Gain/1
  Integrator1/1 -> m_N2_ca/1, MATLAB Function/3(m_N2), Scope2/2
  P_an/1 -> MATLAB Function/1(P_an)
  T_an/1 -> MATLAB Function/2(T_an)
  Constant1/1 -> MATLAB Function/6(R_O2)
  Constant/1 -> MATLAB Function/5(R_N2)
  Integrator/1 -> m_O2_ca/1, Scope2/1, MATLAB Function/4(m_O2)
  Constant2/1 -> Add3/2
  Pipe Volume/1 -> Add3/1
  Add3/1 -> MATLAB Function1/1(V_recirc)
  W_O2_ca_cf/1 -> Gain1/1
  Pulse Generator/1 -> Integrator/2, Integrator1/2
  MATLAB Function1/1(H2_ratio) -> H2_ratio/1, Scope1/1
  Gain/1 -> Integrator1/1
  Gain1/1 -> Integrator/1
  MATLAB Function/1(V_N2) -> MATLAB Function1/2(V_cont)
  MATLAB Function/2(V_O2) -> Scope/1

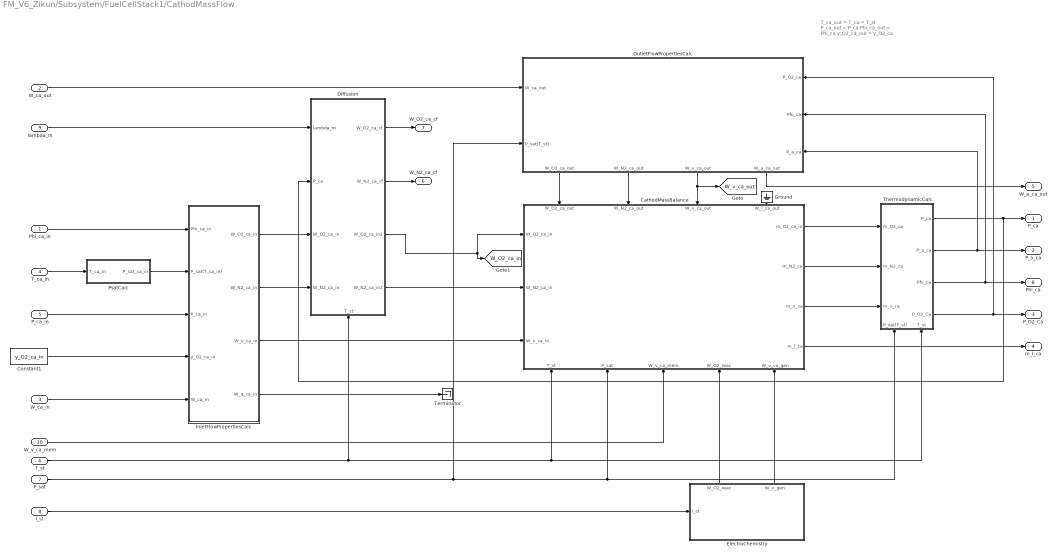
== system FM_V6_Zikun/Subsystem/FuelCellStack1/CathodMassFlow ==
  note: T_ca_out = T_ca = T_st
      | P_ca_out = P_ca
      | Phi_ca_out = Phi_ca
      | y_O2_ca_out = y_O2_ca
  Phi_ca_in : Inport
  W_ca_out : Inport  Port=2
  W_ca_in : Inport  Port=3
  T_ca_in : Inport  Port=4
  P_ca_in : Inport  Port=5
  T_st : Inport  Port=6
  P_sat : Inport  Port=7
  I_st : Inport  Port=8
  lambda_m : Inport  Port=9
  W_v_ca_mem : Inport  Port=10
  CathodMassBalance : Subsystem
      settings: PortSchema="{\"entries\":[{\"content\":{\"sides\":[{\"content\":{\"connectorIds\":[\"In1\",\"In2\",\"In3\"]},\"type\":\"ConnectorPlacement.EquallySpacedRectSide\",\"uuid\":\"630eb789-c97e-4aa4-a033-cf5946298753\"},{\"content\":{\"connectorIds\":[\"Out1\",\"Out2\",\"Out3\",\"Out4\"],\"side\":\"RIGHT\"},\"type\":\"ConnectorPlacement.EquallySpacedRectSide\",\"uuid\":\"61a0dd9e-758e-4b61-90c9-1b16fa21b16a\"},{\"content\":{\"connectorIds\":[\"In4\",\"In5\",\"In6\",\"In7\"],\"side\":\"TOP\"},\"type\":\"ConnectorPlacement.EquallySpacedRectSide\",\"uuid\":\"4e0b935a-479a-4410-a341-3070ed80364f\"},{\"content\":{\"connectorIds\":[\"In8\",\"In9\",\"In10\",\"In11\",\"In12\"],\"side\":\"BOTTOM\"},\"type\":\"ConnectorPlacement.EquallySpacedRectSide\",\"uuid\":\"aa9a69d1-6ace-4a6f-8b04-892854017faa\"}]},\"type\":\"ConnectorPlacement.EquallySpacedConnector\",\"uuid\":\"3f7334b3-e4ed-4b14-8f6e-cfa7bf263ab9\"}],\"packageUris\":[\"http://schema.mathworks.com/mf0/Connector/R2020b\"],\"version\":\"1.0\"}"
  Constant1 : Constant  Value=y_O2_ca_in
  Diffusion : Subsystem
      settings: PortSchema="{\"entries\":[{\"content\":{\"sides\":[{\"content\":{\"connectorIds\":[\"In1\",\"In2\",\"In3\",\"In4\"]},\"type\":\"ConnectorPlacement.EquallySpacedRectSide\",\"uuid\":\"e4477e29-97bf-4f7d-b580-4a3870c95863\"},{\"content\":{\"connectorIds\":[\"Out1\",\"Out2\",\"Out3\",\"Out4\"],\"side\":\"RIGHT\"},\"type\":\"ConnectorPlacement.EquallySpacedRectSide\",\"uuid\":\"f560e4f7-16ea-4bc2-9662-c31ca7e89dcc\"},{\"content\":{\"connectorIds\":[],\"side\":\"TOP\"},\"type\":\"ConnectorPlacement.EquallySpacedRectSide\",\"uuid\":\"52c39bd9-a521-4b0c-a2b4-2ce72e8df433\"},{\"content\":{\"connectorIds\":[\"In5\"],\"side\":\"BOTTOM\"},\"type\":\"ConnectorPlacement.EquallySpacedRectSide\",\"uuid\":\"00bb3f75-7283-4ce4-836a-8a172d1404a2\"}]},\"type\":\"ConnectorPlacement.EquallySpacedConnector\",\"uuid\":\"e836c1df-d3e0-4309-9324-b181a1c7a102\"}],\"packageUris\":[\"http://schema.mathworks.com/mf0/Connector/R2020b\"],\"version\":\"1.0\"}"
  ElectroChemistry : Subsystem
      settings: PortSchema="{\"entries\":[{\"content\":{\"sides\":[{\"content\":{\"connectorIds\":[]},\"type\":\"ConnectorPlacement.EquallySpacedRectSide\",\"uuid\":\"717b8895-0b7f-4e42-9a1b-a5398c6af2de\"},{\"content\":{\"connectorIds\":[\"Out1\",\"Out2\"],\"side\":\"RIGHT\"},\"type\":\"ConnectorPlacement.EquallySpacedRectSide\",\"uuid\":\"543d7451-d141-4e40-b2f0-7c2732f55847\"},{\"content\":{\"connectorIds\":[\"In1\"],\"side\":\"TOP\"},\"type\":\"ConnectorPlacement.EquallySpacedRectSide\",\"uuid\":\"3105341a-b8ba-45de-95b6-94bc2249d195\"}]},\"type\":\"ConnectorPlacement.EquallySpacedConnector\",\"uuid\":\"b4c52fca-680e-41a5-8f0e-b4ed6e03bb02\"}],\"packageUris\":[\"http://schema.mathworks.com/mf0/Connector/R2020b\"],\"version\":\"1.0\"}"
  Ground : Ground
  InletFlowPropertiesCalc : Subsystem
  OutletFlowPropertiesCalc : Subsystem
      settings: PortSchema="{\"entries\":[{\"content\":{\"sides\":[{\"content\":{\"connectorIds\":[]},\"type\":\"ConnectorPlacement.EquallySpacedRectSide\",\"uuid\":\"1ac3cd26-c6f9-4678-a43b-89d74228e3da\"},{\"content\":{\"connectorIds\":[\"Out1\",\"Out2\",\"Out3\",\"Out4\"],\"side\":\"RIGHT\"},\"type\":\"ConnectorPlacement.EquallySpacedRectSide\",\"uuid\":\"e8374325-0971-4eae-996c-945c49276d1a\"},{\"content\":{\"connectorIds\":[\"In1\",\"In2\"],\"side\":\"TOP\"},\"type\":\"ConnectorPlacement.EquallySpacedRectSide\",\"uuid\":\"e1484837-f333-492b-af5c-11e40db9a824\"},{\"content\":{\"connectorIds\":[\"In3\",\"In4\",\"In5\"],\"side\":\"BOTTOM\"},\"type\":\"ConnectorPlacement.EquallySpacedRectSide\",\"uuid\":\"fb6d36b2-de5c-47a1-b852-7eb02f1c301e\"}]},\"type\":\"ConnectorPlacement.EquallySpacedConnector\",\"uuid\":\"58e29f0f-5a8f-42b3-8c0c-a4515a273d1c\"}],\"packageUris\":[\"http://schema.mathworks.com/mf0/Connector/R2020b\"],\"version\":\"1.0\"}"
  PsatCalc : MATLAB Function  TreatAsAtomicUnit=on
  Terminator : Terminator
  ThermodynamicCalc : Subsystem
      settings: PortSchema="{\"entries\":[{\"content\":{\"sides\":[{\"content\":{\"connectorIds\":[\"In1\",\"In2\",\"In3\"]},\"type\":\"ConnectorPlacement.EquallySpacedRectSide\",\"uuid\":\"f2bf2484-4ede-4213-b7af-9058cec10d25\"},{\"content\":{\"connectorIds\":[\"Out1\",\"Out2\",\"Out3\",\"Out4\"],\"side\":\"RIGHT\"},\"type\":\"ConnectorPlacement.EquallySpacedRectSide\",\"uuid\":\"d3102b41-db4e-449f-8ec9-c6089202107d\"},{\"content\":{\"connectorIds\":[],\"side\":\"TOP\"},\"type\":\"ConnectorPlacement.EquallySpacedRectSide\",\"uuid\":\"27559761-62d4-4ec3-b93b-da2f77931cab\"},{\"content\":{\"connectorIds\":[\"In4\",\"In5\"],\"side\":\"BOTTOM\"},\"type\":\"ConnectorPlacement.EquallySpacedRectSide\",\"uuid\":\"8ccd105c-cbb0-45ec-a24a-45224f181c0d\"}]},\"type\":\"ConnectorPlacement.EquallySpacedConnector\",\"uuid\":\"c3e611e3-9464-4b5e-b114-fb5b738a49c3\"}],\"packageUris\":[\"http://schema.mathworks.com/mf0/Connector/R2020b\"],\"version\":\"1.0\"}"
  P_ca : Outport
  P_a_ca : Outport  Port=2
  P_O2_Ca : Outport  Port=3
  m_l_ca : Outport  Port=4
  W_a_ca_out : Outport  Port=5
  W_N2_ca_cf : Outport  Port=6
  W_O2_ca_cf : Outport  Port=7
  Phi_ca : Outport  Port=8
  tag scope: W_O2_ca_in=global, W_v_ca_out=global
  wires:
  ThermodynamicCalc/2(P_a_ca) -> P_a_ca/1, OutletFlowPropertiesCalc/5(P_a_ca)
  ThermodynamicCalc/3(Phi_ca) -> OutletFlowPropertiesCalc/4(Phi_ca), Phi_ca/1
  ThermodynamicCalc/4(P_O2_Ca) -> OutletFlowPropertiesCalc/3(P_O2_ca), P_O2_Ca/1
  CathodMassBalance/1(m_O2_ca_in) -> ThermodynamicCalc/1(m_O2_ca)
  CathodMassBalance/2(m_N2_ca) -> ThermodynamicCalc/2(m_N2_ca)
  CathodMassBalance/3(m_v_ca) -> ThermodynamicCalc/3(m_v_ca)
  InletFlowPropertiesCalc/3(W_v_ca_in) -> CathodMassBalance/3(W_v_ca_in)
  Phi_ca_in/1 -> InletFlowPropertiesCalc/1(Phi_ca_in)
  ElectroChemistry/1(W_O2_reac) -> CathodMassBalance/11(W_O2_reac)
  OutletFlowPropertiesCalc/1(W_O2_ca_out) -> CathodMassBalance/4(W_O2_ca_out)
  OutletFlowPropertiesCalc/2(W_N2_ca_out) -> CathodMassBalance/5(W_N2_ca_out)
  OutletFlowPropertiesCalc/3(W_v_ca_out) -> [W_v_ca_out], CathodMassBalance/6(W_v_ca_out)
  W_ca_out/1 -> OutletFlowPropertiesCalc/1(W_ca_out)
  T_st/1 -> ThermodynamicCalc/5(T_st), CathodMassBalance/8(T_st), Diffusion/5(T_st)
  I_st/1 -> ElectroChemistry/1(I_st)
  P_sat/1 -> OutletFlowPropertiesCalc/2(P_sat(T_st)), ThermodynamicCalc/4(P_sat(T_st)), CathodMassBalance/9(P_sat)
  W_v_ca_mem/1 -> CathodMassBalance/10(W_v_ca_mem)
  W_ca_in/1 -> InletFlowPropertiesCalc/5(W_ca_in)
  Constant1/1 -> InletFlowPropertiesCalc/4(y_O2_ca_in)
  PsatCalc/1(P_sat_ca_in) -> InletFlowPropertiesCalc/2(P_sat(T_ca_in))
  OutletFlowPropertiesCalc/4(W_a_ca_out) -> W_a_ca_out/1
  CathodMassBalance/4(m_l_ca) -> m_l_ca/1
  InletFlowPropertiesCalc/4(W_a_ca_in) -> Terminator/1
  Ground/1 -> CathodMassBalance/7(W_l_ca_out)
  T_ca_in/1 -> PsatCalc/1(T_ca_in)
  ThermodynamicCalc/1(P_ca) -> Diffusion/2(P_ca), P_ca/1
  ElectroChemistry/2(W_v_gen) -> CathodMassBalance/12(W_v_ca_gen)
  Diffusion/3(W_O2_ca_in2) -> CathodMassBalance/1(W_O2_ca_in), [W_O2_ca_in]
  Diffusion/4(W_N2_ca_in2) -> CathodMassBalance/2(W_N2_ca_in)
  InletFlowPropertiesCalc/1(W_O2_ca_in) -> Diffusion/3(W_O2_ca_in)
  InletFlowPropertiesCalc/2(W_N2_ca_in) -> Diffusion/4(W_N2_ca_in)
  P_ca_in/1 -> InletFlowPropertiesCalc/3(P_ca_in)
  Diffusion/1(W_O2_ca_cf) -> W_O2_ca_cf/1
  Diffusion/2(W_N2_ca_cf) -> W_N2_ca_cf/1
  lambda_m/1 -> Diffusion/1(lambda_m)
